simulink model "sampleModel232"  (R2021b)
settings: Solver=VariableStepAuto  StartTime=0.0  StopTime=10.0  RelTol=1e-3
undefined symbols (not defined in the file or in its folder): Newton, Raphson
libraries: simulink x12, slpidlib x3
settings Model: Creator=user  LastModifiedBy=user

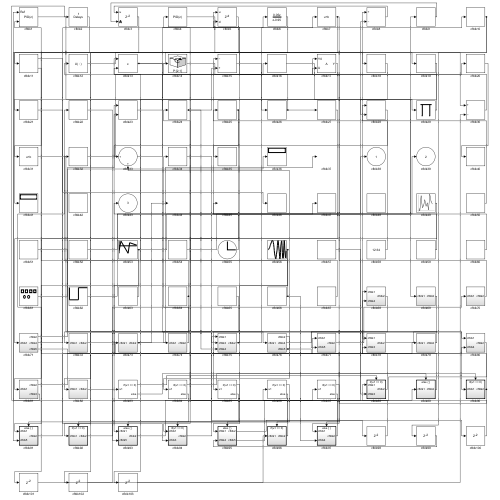
[thumbnail: Simulink's stored preview of the top-level diagram]
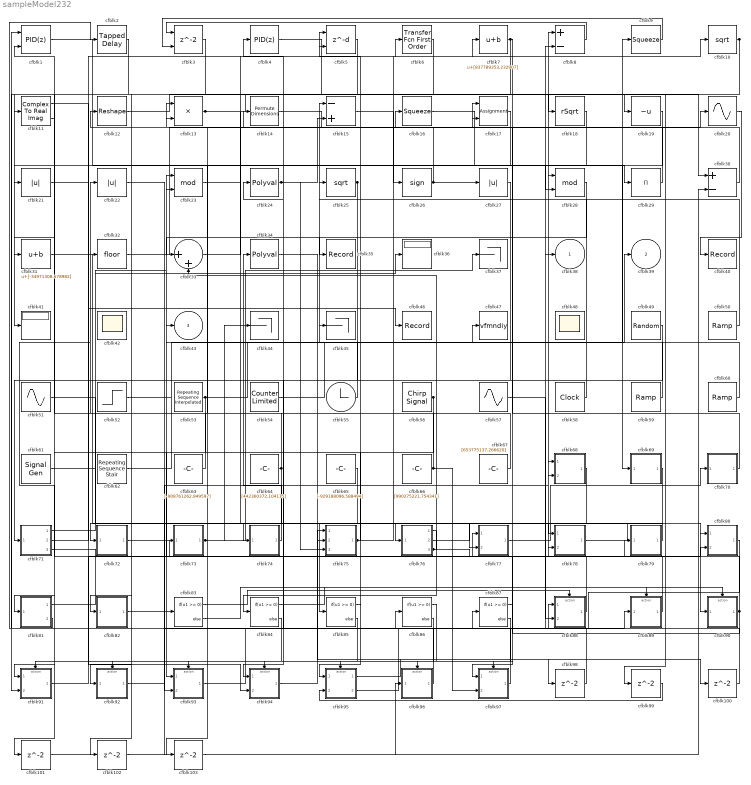
== system sampleModel232 ==
  cfblk1 : slpidlib/PID Controller (2DOF)  Controller=PID  Form=Parallel  TimeDomain=Discrete-time  UseExternalTs=off  SampleTime=1  IntegratorMethod=Forward Euler  FilterMethod=Forward Euler  ControllerParametersSource=internal  P=1  I=1  D=0  UseFilter=on  N=100  b=1  c=1  TunerSelectOption=Transfer Function Based (PID Tuner App)  InitialConditionSource=internal  InitialConditionForIntegrator=0  InitialConditionForFilter=0  DifferentiatorICPrevScaledInput=0  ExternalReset=none  TrackingMode=off  Kt=1  LimitOutput=off  SatLimitsSource=internal  UpperSaturationLimit=inf  LowerSaturationLimit=-inf  LinearizeAsGain=off  AntiWindupMode=none  Kb=1  POutMin=[]  POutMax=[]  IOutMin=[]  IOutMax=[]  DOutMin=[]  DOutMax=[]  NOutMin=[]  NOutMax=[]  bOutMin=[]  bOutMax=[]  cOutMin=[]  cOutMax=[]  SumOutMin=[]  SumOutMax=[]  SaturationOutMin=[]  SaturationOutMax=[]  PParamMin=[]  PParamMax=[]  IParamMin=[]  IParamMax=[]  DParamMin=[]  DParamMax=[]  NParamMin=[]  NParamMax=[]  bParamMin=[]  bParamMax=[]  cParamMin=[]  cParamMax=[]  KbParamMin=[]  KbParamMax=[]  KtParamMin=[]  KtParamMax=[]  KbOutMin=[]  KbOutMax=[]  KtOutMin=[]  KtOutMax=[]  IntegratorOutMin=[]  IntegratorOutMax=[]  FilterOutMin=[]  FilterOutMax=[]  SumI1OutMin=[]  SumI1OutMax=[]  SumI2OutMin=[]  SumI2OutMax=[]  SumI3OutMin=[]  SumI3OutMax=[]  SumI4OutMin=[]  SumI4OutMax=[]  SumDOutMin=[]  SumDOutMax=[]  Sum1OutMin=[]  Sum1OutMax=[]  Sum2OutMin=[]  Sum2OutMax=[]  Sum3OutMin=[]  Sum3OutMax=[]  DifferentiatorOutMin=[]  DifferentiatorOutMax=[]  FilterDiffOutCoefMin=[]  FilterDiffOutCoefMax=[]  ReciprocalOutMin=[]  ReciprocalOutMax=[]  SumDenOutMin=[]  SumDenOutMax=[]  SumNumOutMin=[]  SumNumOutMax=[]  DivideOutMin=[]  DivideOutMax=[]  UdiffTsProdOutMin=[]  UdiffTsProdOutMax=[]  NTsProdOutMin=[]  NTsProdOutMax=[]  UintegralTsProdOutMin=[]  UintegralTsProdOutMax=[]  UngainTsProdOutMin=[]  UngainTsProdOutMax=[]  IntegratorContinuousStateAttributes=''  IntegratorStateMustResolveToSignalObject=off  IntegratorRTWStateStorageClass=Auto  FilterContinuousStateAttributes=''  FilterStateMustResolveToSignalObject=off  FilterRTWStateStorageClass=Auto  ParallelPVariant=InternalParameters  IdealPVariant=Disabled  IVariant=InternalParameters  DVariant=InternalParameters  bVariant=InternalParameters  cVariant=InternalParameters  IntegratorVariant=Discrete  SatVariant=Disabled  AWVariant=Passthrough  PCopyVariant=Disabled  TRVariant=Disabled  FdbkBlocksVariant=Forward  IdealPFdbkVariant=Disabled  SatFdbkVariant=Disabled  DerivativeFilterVariant=ForwardEulerFilter  NVariant=InternalParameters  NCopyVariant=Disabled  FilterICVariant=InternalICsFilter  IntegratorICVariant=InternalICs  ExternalResetVariant=Disabled  TRSumVariant=Passthrough  SumFdbkVariant=Disabled  SumVariant=Sum_PID  TsampFilterVariant=InternalTs  TsampNgainVariant=Passthrough  TsampIntegralVariant=Passthrough  ExternalSaturationOutDataTypeStr=Inherit: Same as second input
      settings: SourceProductBaseCode=SL
  cfblk10 : Sqrt  SaturateOnIntegerOverflow=on
  cfblk{98..103} (6 alike) : Delay  SampleTime=1
  cfblk11 : ComplexToRealImag
  cfblk12 : Reshape
  cfblk13 : Product
  cfblk14 : PermuteDimensions
  cfblk15 : Sum  Inputs=-+
  cfblk16 : Squeeze
  cfblk17 : Assignment  DiagnosticForDimensions=Warning  IndexOptions=Index vector (dialog)  Indices=1  OutputSizes=1
  cfblk18 : Sqrt  Operator=rSqrt  AlgorithmType=Newton-Raphson  SaturateOnIntegerOverflow=on
  cfblk19 : UnaryMinus
  cfblk2 : simulink/Discrete/Tapped Delay  vinit=0.0  samptime=-1  NumDelays=1  DelayOrder=Oldest  includeCurrent=off
  cfblk20 : Sin  TimeSource=Use external signal  SampleTime=0
  cfblk21 : Abs
  cfblk22 : Abs
  cfblk23 : Math  Operator=mod  SaturateOnIntegerOverflow=on
  cfblk24 : Polyval  Coefs=[ +2.081618890e-019, -1.441693666e-014, +4.719686976e-010, -8.536869453e-006, +1.621573104e-001, -8.087801117e+001 ]
  cfblk25 : Sqrt  SaturateOnIntegerOverflow=on
  cfblk26 : Signum
  cfblk27 : Abs
  cfblk28 : Math  Operator=mod  SaturateOnIntegerOverflow=on
  cfblk29 : Product  Inputs=*
  cfblk3 : Delay  ShowEnablePort=on  SampleTime=1
      settings: InputPortMap=u0,e6
  cfblk30 : Sum  Inputs=+-
  cfblk31 : Bias  Bias=[-34971308.678982]
  cfblk32 : Rounding
  cfblk33 : Sum  Inputs=|++
  cfblk34 : Polyval  Coefs=[ +2.081618890e-019, -1.441693666e-014, +4.719686976e-010, -8.536869453e-006, +1.621573104e-001, -8.087801117e+001 ]
  cfblk35 : Record  FileSettingsInternal="{\"entries\":[{\"content\":{\"excelSettings\":{\"content\":{},\"type\":\"Streamout.ExcelSettings\"}},\"type\":\"Streamout.FileSettingStorage\",\"uuid\":\"16fe7588-171d-4433-9593-ebc7fb32ed17\"}],\"packageUris\":[\"http://schema.mathworks.com/mf0/streamout_blocks/R2020a\"],\"version\":\"1.0\"}"  SignalsInternal="{\"entries\":[{\"content\":{\"signals\":[{\"content\":{\"blockPath\":[\"sampleModel232/cfblk35\"],\"channel\":[],\"dimensions\":[1],\"domain\":\"sampleModel232/cfblk35\",\"lineColor\":\"#ff6929\",\"plots\":[1],\"port\":1,\"sid\":[\"\"],\"signalID\":9135,\"signalName\":\"cfblk25\"},\"type\":\"RecordBlkView.Signal\",\"uuid\":\"2eec1ae0-d335-4178-83e4-c7d2b4e411f4\"}]},\"type\":\"RecordBlkView.InputSignals\",\"uuid\":\"9f3df593-7b50-41bb-8005-8753dcf3348f\"}],\"packageUris\":[\"http://schema.mathworks.com/mf0/streamout_blocks/R2020a\"],\"version\":\"1.0\"}"  VisualizationBindings="{\"sparklinesplugin\":{\"info\":[{\"bindingParametersList\":[],\"subplotID\":1}]}}"
  cfblk36 : Display
  cfblk37 : Terminator
  cfblk4 : slpidlib/PID Controller  Controller=PID  Form=Parallel  TimeDomain=Discrete-time  UseExternalTs=off  SampleTime=1  IntegratorMethod=Forward Euler  FilterMethod=Forward Euler  ControllerParametersSource=internal  P=1  I=1  D=0  UseFilter=on  N=100  TunerSelectOption=Transfer Function Based (PID Tuner App)  InitialConditionSource=internal  InitialConditionForIntegrator=0  InitialConditionForFilter=0  DifferentiatorICPrevScaledInput=0  ExternalReset=none  TrackingMode=off  Kt=1  LimitOutput=off  SatLimitsSource=internal  UpperSaturationLimit=inf  LowerSaturationLimit=-inf  LinearizeAsGain=off  AntiWindupMode=none  Kb=1  POutMin=[]  POutMax=[]  IOutMin=[]  IOutMax=[]  DOutMin=[]  DOutMax=[]  NOutMin=[]  NOutMax=[]  SumOutMin=[]  SumOutMax=[]  SaturationOutMin=[]  SaturationOutMax=[]  PParamMin=[]  PParamMax=[]  IParamMin=[]  IParamMax=[]  DParamMin=[]  DParamMax=[]  NParamMin=[]  NParamMax=[]  KbParamMin=[]  KbParamMax=[]  KtParamMin=[]  KtParamMax=[]  KbOutMin=[]  KbOutMax=[]  KtOutMin=[]  KtOutMax=[]  IntegratorOutMin=[]  IntegratorOutMax=[]  FilterOutMin=[]  FilterOutMax=[]  SumI1OutMin=[]  SumI1OutMax=[]  SumI2OutMin=[]  SumI2OutMax=[]  SumI3OutMin=[]  SumI3OutMax=[]  SumI4OutMin=[]  SumI4OutMax=[]  SumDOutMin=[]  SumDOutMax=[]  DifferentiatorOutMin=[]  DifferentiatorOutMax=[]  FilterDiffOutCoefMin=[]  FilterDiffOutCoefMax=[]  ReciprocalOutMin=[]  ReciprocalOutMax=[]  SumDenOutMin=[]  SumDenOutMax=[]  SumNumOutMin=[]  SumNumOutMax=[]  DivideOutMin=[]  DivideOutMax=[]  UdiffTsProdOutMin=[]  UdiffTsProdOutMax=[]  NTsProdOutMin=[]  NTsProdOutMax=[]  UintegralTsProdOutMin=[]  UintegralTsProdOutMax=[]  UngainTsProdOutMin=[]  UngainTsProdOutMax=[]  IntegratorContinuousStateAttributes=''  IntegratorStateMustResolveToSignalObject=off  IntegratorRTWStateStorageClass=Auto  FilterContinuousStateAttributes=''  FilterStateMustResolveToSignalObject=off  FilterRTWStateStorageClass=Auto  ParallelPVariant=InternalParameters  IdealPVariant=Disabled  IVariant=InternalParameters  DVariant=InternalParameters  IntegratorVariant=Discrete  SatVariant=Disabled  AWVariant=Passthrough  PCopyVariant=Disabled  TRVariant=Disabled  FdbkBlocksVariant=Forward  IdealPFdbkVariant=Disabled  SatFdbkVariant=Disabled  DerivativeFilterVariant=ForwardEulerFilter  NVariant=InternalParameters  NCopyVariant=Disabled  FilterICVariant=InternalICsFilter  IntegratorICVariant=InternalICs  ExternalResetVariant=Disabled  TRSumVariant=Passthrough  SumFdbkVariant=Disabled  SumVariant=Sum_PID  TsampFilterVariant=InternalTs  TsampNgainVariant=Passthrough  TsampIntegralVariant=Passthrough  ExternalSaturationOutDataTypeStr=Inherit: Same as second input
  cfblk40 : Record  FileSettingsInternal="{\"entries\":[{\"content\":{\"excelSettings\":{\"content\":{},\"type\":\"Streamout.ExcelSettings\"}},\"type\":\"Streamout.FileSettingStorage\",\"uuid\":\"38fde572-acd1-41f4-bd4f-f8c5a046ea04\"}],\"packageUris\":[\"http://schema.mathworks.com/mf0/streamout_blocks/R2020a\"],\"version\":\"1.0\"}"  SignalsInternal="{\"entries\":[{\"content\":{\"signals\":[{\"content\":{\"blockPath\":[\"sampleModel232/cfblk40\"],\"channel\":[],\"dimensions\":[1,1],\"domain\":\"sampleModel232/cfblk40\",\"lineColor\":\"#b746ff\",\"plots\":[1],\"port\":1,\"sid\":[\"\"],\"signalID\":9139,\"signalName\":\"cfblk20\"},\"type\":\"RecordBlkView.Signal\",\"uuid\":\"00039949-2aab-479e-a4e6-845a35bec5f1\"}]},\"type\":\"RecordBlkView.InputSignals\",\"uuid\":\"6f56bbc5-1270-4389-943e-16f85e3705aa\"}],\"packageUris\":[\"http://schema.mathworks.com/mf0/streamout_blocks/R2020a\"],\"version\":\"1.0\"}"  VisualizationBindings="{\"sparklinesplugin\":{\"info\":[{\"bindingParametersList\":[],\"subplotID\":1}]}}"
  cfblk41 : Display
  cfblk42 : Scope
      settings: Floating=on
  cfblk44 : Terminator
  cfblk45 : Terminator
  cfblk46 : Record  FileSettingsInternal="{\"entries\":[{\"content\":{\"excelSettings\":{\"content\":{},\"type\":\"Streamout.ExcelSettings\"}},\"type\":\"Streamout.FileSettingStorage\",\"uuid\":\"14fcbd9d-bac8-4dc1-8b82-4cc51f23d5c0\"}],\"packageUris\":[\"http://schema.mathworks.com/mf0/streamout_blocks/R2020a\"],\"version\":\"1.0\"}"  SignalsInternal="{\"entries\":[{\"content\":{\"signals\":[{\"content\":{\"blockPath\":[\"sampleModel232/cfblk46\"],\"channel\":[],\"dimensions\":[1],\"domain\":\"sampleModel232/cfblk46\",\"lineColor\":\"#64d413\",\"plots\":[1],\"port\":1,\"sid\":[\"\"],\"signalID\":9143,\"signalName\":\"cfblk21\"},\"type\":\"RecordBlkView.Signal\",\"uuid\":\"5c7e960c-d979-495a-80ca-2dc05e47916f\"}]},\"type\":\"RecordBlkView.InputSignals\",\"uuid\":\"40783f06-613e-4da5-a4b1-e85038e253b6\"}],\"packageUris\":[\"http://schema.mathworks.com/mf0/streamout_blocks/R2020a\"],\"version\":\"1.0\"}"  VisualizationBindings="{\"sparklinesplugin\":{\"info\":[{\"bindingParametersList\":[],\"subplotID\":1}]}}"
  cfblk47 : ToWorkspace  VariableName=vfmndiy  SaveFormat=Timeseries  SampleTime=-1
  cfblk48 : Scope
      settings: Floating=on
  cfblk49 : UniformRandomNumber  Minimum=[-6531070159.920979]  Maximum=[9416126796.491138]  Seed=[69575523.000000]  SampleTime=0.1
  cfblk5 : Delay  DelayLengthSource=Input port  SampleTime=1
      settings: InputPortMap=u0,p1
  cfblk50 : simulink/Sources/Ramp  slope=[4184.454885]  start=[6.485913]  InitialOutput=[-74727.507145]
  cfblk51 : Sin  Amplitude=[660836830.199607]  Bias=[-337757806.375018]  SampleTime=0
  cfblk52 : Step  Time=[5.000000]  Before=[-35343837.291775]  After=[252133215.622026]  SampleTime=0
  cfblk53 : simulink/Sources/Repeating Sequence Interpolated  OutValues=[-608474345.099651, 600750965.712178, -937019260.295574, 395421429.511669, 62724602.129927]  TimeValues=[0 0.1 0.5 0.6 1].'  LookUpMeth=Use Input Nearest  tsamp=0.01  OutMin=[]  OutMax=[]  OutDataTypeStr=double  OutputDataTypeScalingMode=double  OutDataType=fixdt(0,8)  OutScaling=2^-10
  cfblk54 : simulink/Sources/Counter Limited  uplimit=[972.000000]  tsamp=-1
  cfblk55 : Clock
  cfblk56 : simulink/Sources/Chirp Signal  f1=[693040230.893386]  T=[-954068434.723357]  f2=[440264525.580880]
  cfblk57 : Sin  Amplitude=[242398372.769042]  Bias=[-91557625.579191]  SampleTime=0
  cfblk58 : DigitalClock
  cfblk59 : simulink/Sources/Ramp  slope=[-2546.341926]  start=[42.940837]  InitialOutput=[85456.918495]
  cfblk6 : simulink/Discrete/Transfer Fcn First Order  PoleZ=0.95  ICPrevOutput=0.0  DoSatur=off
  cfblk60 : simulink/Sources/Ramp  slope=[-9968.943757]  start=[29.827868]  InitialOutput=[-927129.818400]
  cfblk61 : SignalGenerator  WaveForm=square  Amplitude=[-206501216.018369]
  cfblk62 : simulink/Sources/Repeating Sequence Stair  OutValues=[-478930033.945131, -287515944.626940]  tsamp=-1  OutMin=[]  OutMax=[]  OutDataTypeStr=double  OutputDataTypeScalingMode=double  OutDataType=fixdt(0,8)  ConRadixGroup=Best Precision: Vector-wise  OutScaling=2^-12
  cfblk63 : Constant  Value=[-908761262.849597]  SampleTime=1
  cfblk64 : Constant  Value=[442360372.104115]  SampleTime=1
  cfblk65 : Constant  Value=[-929188096.588494]  SampleTime=1
  cfblk66 : Constant  Value=[990275221.754341]  SampleTime=1
  cfblk67 : Constant  Value=[653775137.266620]  SampleTime=1
  cfblk68 : Subsystem
  cfblk69 : Subsystem
  cfblk7 : Bias  Bias=[837789353.232907]
  cfblk70 : Subsystem
  cfblk71 : Subsystem
  cfblk72 : Subsystem
  cfblk73 : Subsystem
  cfblk74 : Subsystem
  cfblk75 : Subsystem
  cfblk76 : Subsystem
  cfblk77 : Subsystem
  cfblk78 : Subsystem
  cfblk79 : Subsystem
  cfblk8 : Sum  Inputs=+-
  cfblk80 : Subsystem
  cfblk81 : Subsystem
  cfblk82 : Subsystem
  cfblk{83..87} (5 alike) : If  IfExpression=u1 >= 0  SampleTime=1
  cfblk88 : Subsystem  TreatAsAtomicUnit=on
  cfblk89 : Subsystem  TreatAsAtomicUnit=on
  cfblk9 : Squeeze
  cfblk90 : Subsystem  TreatAsAtomicUnit=on
  cfblk91 : Subsystem  TreatAsAtomicUnit=on
  cfblk92 : Subsystem  TreatAsAtomicUnit=on
  cfblk93 : Subsystem  TreatAsAtomicUnit=on
  cfblk94 : Subsystem  TreatAsAtomicUnit=on
  cfblk95 : Subsystem  TreatAsAtomicUnit=on
  cfblk96 : Subsystem  TreatAsAtomicUnit=on
  cfblk97 : Subsystem  TreatAsAtomicUnit=on
  cfblk38 : Outport
  cfblk39 : Outport  Port=2
  cfblk43 : Outport  Port=3
  wires:
  cfblk32/1 -> cfblk16/1
  cfblk61/1 -> cfblk36/1
  cfblk93/1(cfblk2) -> cfblk87/1
  cfblk88/1(cfblk2) -> cfblk8/1
  cfblk80/1(cfblk2) -> cfblk88/1(cfblk1)
  cfblk79/1(cfblk2) -> cfblk72/1(cfblk1)
  cfblk12/1 -> cfblk18/1
  cfblk50/1 -> cfblk15/1
  cfblk90/1(cfblk2) -> cfblk22/1, cfblk78/2(cfblk3)
  cfblk51/1 -> cfblk90/1(cfblk1)
  cfblk89/1(cfblk2) -> cfblk23/1
  cfblk14/1 -> cfblk20/1
  cfblk17/1 -> cfblk41/1
  cfblk27/1 -> cfblk71/1(cfblk1)
  cfblk54/1 -> cfblk8/2
  cfblk52/1 -> cfblk47/1
  cfblk8/1 -> cfblk3/1
  cfblk64/1 -> cfblk92/1(cfblk1), cfblk1/2
  cfblk53/1 -> cfblk93/1(cfblk1), cfblk39/1
  cfblk74/1(cfblk2) -> cfblk34/1
  cfblk97/1(cfblk2) -> cfblk24/1
  cfblk26/1 -> cfblk27/1, cfblk5/1
  cfblk65/1 -> cfblk85/1
  cfblk60/1 -> cfblk25/1
  cfblk92/1(cfblk2) -> cfblk89/1(cfblk1)
  cfblk15/1 -> cfblk26/1
  cfblk24/1 -> cfblk15/2, cfblk75/3(cfblk4)
  cfblk31/1 -> cfblk76/1(cfblk1)
  cfblk7/1 -> cfblk21/1, cfblk97/1(cfblk1)
  cfblk4/1 -> cfblk30/1
  cfblk55/1 -> cfblk45/1
  cfblk66/1 -> cfblk4/1, cfblk97/2(cfblk4)
  cfblk56/1 -> cfblk91/1(cfblk1), cfblk95/1(cfblk1)
  cfblk78/1(cfblk2) -> cfblk80/1(cfblk1)
  cfblk21/1 -> cfblk46/1
  cfblk20/1 -> cfblk40/1
  cfblk33/1 -> cfblk7/1
  cfblk13/1 -> cfblk19/1, cfblk75/2(cfblk3)
  cfblk1/1 -> cfblk29/1
  cfblk30/1 -> cfblk12/1
  cfblk57/1 -> cfblk88/2(cfblk3)
  cfblk81/1(cfblk2) -> cfblk68/1(cfblk1)
  cfblk96/1(cfblk2) -> cfblk14/1
  cfblk91/1(cfblk2) -> cfblk77/1(cfblk1)
  cfblk75/1(cfblk2) -> cfblk10/1, cfblk5/2
  cfblk73/1(cfblk2) -> cfblk37/1, cfblk44/1
  cfblk94/1(cfblk2) -> cfblk75/1(cfblk1)
  cfblk58/1 -> cfblk28/1
  cfblk81/2(cfblk3) -> cfblk2/1
  cfblk71/1(cfblk2) -> cfblk23/2
  cfblk9/1 -> cfblk3/2
  cfblk76/1(cfblk2) -> cfblk84/1
  cfblk5/1 -> cfblk91/2(cfblk5)
  cfblk6/1 -> cfblk11/1
  cfblk77/1(cfblk2) -> cfblk70/1(cfblk1)
  cfblk68/1(cfblk2) -> cfblk74/1(cfblk1)
  cfblk63/1 -> cfblk32/1
  cfblk82/1(cfblk2) -> cfblk68/2(cfblk4)
  cfblk25/1 -> cfblk81/1(cfblk1), cfblk35/1
  cfblk16/1 -> cfblk69/1(cfblk1)
  cfblk62/1 -> cfblk9/1
  cfblk49/1 -> cfblk94/1(cfblk1)
  cfblk67/1 -> cfblk13/1
  cfblk59/1 -> cfblk43/1
  cfblk22/1 -> cfblk93/2(cfblk5)
  cfblk10/1 -> cfblk82/1(cfblk1), cfblk99/1
  cfblk2/1 -> cfblk31/1
  cfblk69/1(cfblk2) -> cfblk77/2(cfblk5)
  cfblk11/1 -> cfblk94/2(cfblk3)
  cfblk19/1 -> cfblk28/2
  cfblk95/2(cfblk5) -> cfblk38/1
  cfblk76/2(cfblk4) -> cfblk78/1(cfblk1)
  cfblk29/1 -> cfblk13/2
  cfblk70/1(cfblk2) -> cfblk17/1
  cfblk76/3(cfblk5) -> cfblk79/1(cfblk1), cfblk33/2
  cfblk72/1(cfblk2) -> cfblk80/2(cfblk4)
  cfblk23/1 -> cfblk17/2
  cfblk71/2(cfblk4) -> cfblk6/1
  cfblk28/1 -> cfblk33/1
  cfblk71/3(cfblk5) -> cfblk73/1(cfblk1)
  cfblk83/1 -> cfblk88/Action
  cfblk83/2 -> cfblk89/Action
  cfblk84/1 -> cfblk90/Action
  cfblk84/2 -> cfblk91/Action
  cfblk85/1 -> cfblk92/Action
  cfblk85/2 -> cfblk93/Action
  cfblk86/1 -> cfblk94/Action
  cfblk86/2 -> cfblk95/Action
  cfblk87/1 -> cfblk96/Action
  cfblk87/2 -> cfblk97/Action
  cfblk34/1 -> cfblk98/1
  cfblk98/1 -> cfblk1/1
  cfblk99/1 -> cfblk95/2(cfblk4)
  cfblk95/1(cfblk2) -> cfblk100/1
  cfblk100/1 -> cfblk86/1
  cfblk11/2 -> cfblk101/1
  cfblk101/1 -> cfblk96/1(cfblk1)
  cfblk3/1 -> cfblk102/1
  cfblk102/1 -> cfblk83/1
  cfblk18/1 -> cfblk103/1
  cfblk103/1 -> cfblk30/2

== system sampleModel232/cfblk68 ==
  cfblk1 : Inport
  cfblk4 : Inport  Port=2
  cfblk3 : simulink/Discrete/Tapped Delay  vinit=0.0  samptime=-1  NumDelays=1  DelayOrder=Oldest  includeCurrent=off
  cfblk2 : Outport
  wires:
  cfblk1/1 -> cfblk3/1
  cfblk3/1 -> cfblk2/1

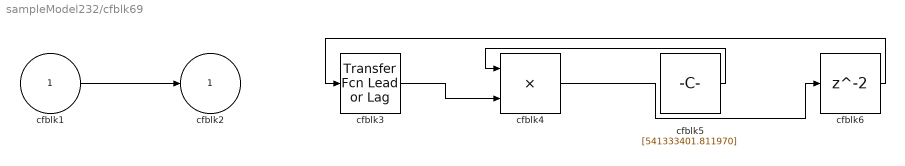
== system sampleModel232/cfblk69 ==
  cfblk1 : Inport
  cfblk3 : simulink/Discrete/Transfer Fcn Lead or Lag  PoleZ=0.95  ZeroZ=0.75  ICPrevOutput=0.0  ICPrevInput=0.0  DoSatur=off
      settings: SourceProductBaseCode=SL
  cfblk4 : Product
  cfblk5 : Constant  Value=[541333401.811970]  SampleTime=1
  cfblk6 : Delay  SampleTime=1
  cfblk2 : Outport
  wires:
  cfblk5/1 -> cfblk4/1
  cfblk1/1 -> cfblk2/1
  cfblk3/1 -> cfblk4/2
  cfblk4/1 -> cfblk6/1
  cfblk6/1 -> cfblk3/1

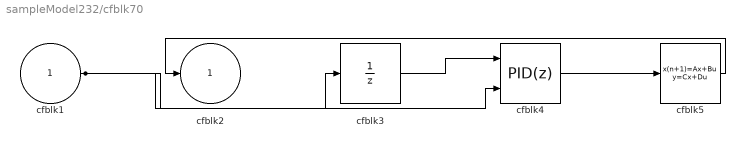
== system sampleModel232/cfblk70 ==
  cfblk1 : Inport
  cfblk3 : UnitDelay  HasFrameUpgradeWarning=on
  cfblk4 : slpidlib/PID Controller (2DOF)  Controller=PID  Form=Parallel  TimeDomain=Discrete-time  UseExternalTs=off  SampleTime=1  IntegratorMethod=Forward Euler  FilterMethod=Forward Euler  ControllerParametersSource=internal  P=1  I=1  D=0  UseFilter=on  N=100  b=1  c=1  TunerSelectOption=Transfer Function Based (PID Tuner App)  InitialConditionSource=internal  InitialConditionForIntegrator=0  InitialConditionForFilter=0  DifferentiatorICPrevScaledInput=0  ExternalReset=none  TrackingMode=off  Kt=1  LimitOutput=off  SatLimitsSource=internal  UpperSaturationLimit=inf  LowerSaturationLimit=-inf  LinearizeAsGain=off  AntiWindupMode=none  Kb=1  POutMin=[]  POutMax=[]  IOutMin=[]  IOutMax=[]  DOutMin=[]  DOutMax=[]  NOutMin=[]  NOutMax=[]  bOutMin=[]  bOutMax=[]  cOutMin=[]  cOutMax=[]  SumOutMin=[]  SumOutMax=[]  SaturationOutMin=[]  SaturationOutMax=[]  PParamMin=[]  PParamMax=[]  IParamMin=[]  IParamMax=[]  DParamMin=[]  DParamMax=[]  NParamMin=[]  NParamMax=[]  bParamMin=[]  bParamMax=[]  cParamMin=[]  cParamMax=[]  KbParamMin=[]  KbParamMax=[]  KtParamMin=[]  KtParamMax=[]  KbOutMin=[]  KbOutMax=[]  KtOutMin=[]  KtOutMax=[]  IntegratorOutMin=[]  IntegratorOutMax=[]  FilterOutMin=[]  FilterOutMax=[]  SumI1OutMin=[]  SumI1OutMax=[]  SumI2OutMin=[]  SumI2OutMax=[]  SumI3OutMin=[]  SumI3OutMax=[]  SumI4OutMin=[]  SumI4OutMax=[]  SumDOutMin=[]  SumDOutMax=[]  Sum1OutMin=[]  Sum1OutMax=[]  Sum2OutMin=[]  Sum2OutMax=[]  Sum3OutMin=[]  Sum3OutMax=[]  DifferentiatorOutMin=[]  DifferentiatorOutMax=[]  FilterDiffOutCoefMin=[]  FilterDiffOutCoefMax=[]  ReciprocalOutMin=[]  ReciprocalOutMax=[]  SumDenOutMin=[]  SumDenOutMax=[]  SumNumOutMin=[]  SumNumOutMax=[]  DivideOutMin=[]  DivideOutMax=[]  UdiffTsProdOutMin=[]  UdiffTsProdOutMax=[]  NTsProdOutMin=[]  NTsProdOutMax=[]  UintegralTsProdOutMin=[]  UintegralTsProdOutMax=[]  UngainTsProdOutMin=[]  UngainTsProdOutMax=[]  IntegratorContinuousStateAttributes=''  IntegratorStateMustResolveToSignalObject=off  IntegratorRTWStateStorageClass=Auto  FilterContinuousStateAttributes=''  FilterStateMustResolveToSignalObject=off  FilterRTWStateStorageClass=Auto  ParallelPVariant=InternalParameters  IdealPVariant=Disabled  IVariant=InternalParameters  DVariant=InternalParameters  bVariant=InternalParameters  cVariant=InternalParameters  IntegratorVariant=Discrete  SatVariant=Disabled  AWVariant=Passthrough  PCopyVariant=Disabled  TRVariant=Disabled  FdbkBlocksVariant=Forward  IdealPFdbkVariant=Disabled  SatFdbkVariant=Disabled  DerivativeFilterVariant=ForwardEulerFilter  NVariant=InternalParameters  NCopyVariant=Disabled  FilterICVariant=InternalICsFilter  IntegratorICVariant=InternalICs  ExternalResetVariant=Disabled  TRSumVariant=Passthrough  SumFdbkVariant=Disabled  SumVariant=Sum_PID  TsampFilterVariant=InternalTs  TsampNgainVariant=Passthrough  TsampIntegralVariant=Passthrough  ExternalSaturationOutDataTypeStr=Inherit: Same as second input
      settings: SourceProductBaseCode=SL
  cfblk5 : DiscreteStateSpace
  cfblk2 : Outport
  wires:
  cfblk5/1 -> cfblk2/1
  cfblk1/1 -> cfblk3/1, cfblk4/2
  cfblk3/1 -> cfblk4/1
  cfblk4/1 -> cfblk5/1

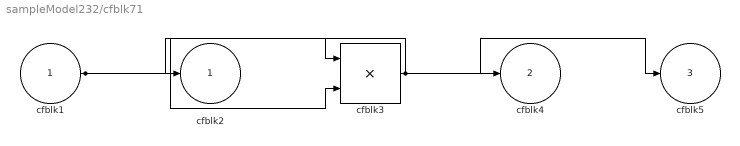
== system sampleModel232/cfblk71 ==
  cfblk1 : Inport
  cfblk3 : Product
  cfblk2 : Outport
  cfblk4 : Outport  Port=2
  cfblk5 : Outport  Port=3
  wires:
  cfblk3/1 -> cfblk4/1, cfblk2/1, cfblk5/1
  cfblk1/1 -> cfblk3/1, cfblk3/2

== system sampleModel232/cfblk72 ==
  cfblk1 : Inport
  cfblk3 : Delay  SampleTime=1
  cfblk2 : Outport
  wires:
  cfblk1/1 -> cfblk3/1
  cfblk3/1 -> cfblk2/1

== system sampleModel232/cfblk73 ==
  cfblk1 : Inport
  cfblk3 : Delay  ShowEnablePort=on  SampleTime=1
      settings: InputPortMap=u0,e6
  cfblk4 : Sqrt  SaturateOnIntegerOverflow=on
  cfblk2 : Outport
  wires:
  cfblk1/1 -> cfblk4/1, cfblk3/2
  cfblk4/1 -> cfblk3/1
  cfblk3/1 -> cfblk2/1

== system sampleModel232/cfblk74 ==
  cfblk1 : Inport
  cfblk3 : Constant  Value=[667065563.085386]  SampleTime=1
  cfblk2 : Outport
  wires:
  cfblk1/1 -> cfblk2/1

== system sampleModel232/cfblk75 ==
  cfblk1 : Inport
  cfblk3 : Inport  Port=2
  cfblk4 : Inport  Port=3
  cfblk2 : Outport
  wires:
  cfblk1/1 -> cfblk2/1

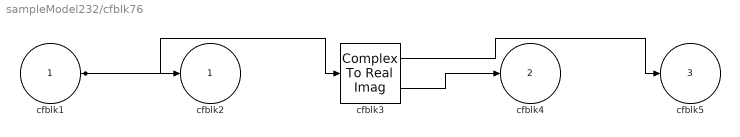
== system sampleModel232/cfblk76 ==
  cfblk1 : Inport
  cfblk3 : ComplexToRealImag
  cfblk2 : Outport
  cfblk4 : Outport  Port=2
  cfblk5 : Outport  Port=3
  wires:
  cfblk3/1 -> cfblk5/1
  cfblk1/1 -> cfblk2/1, cfblk3/1
  cfblk3/2 -> cfblk4/1

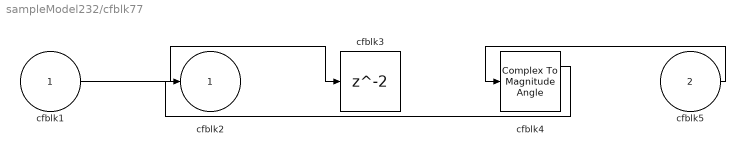
== system sampleModel232/cfblk77 ==
  cfblk1 : Inport
  cfblk5 : Inport  Port=2
  cfblk3 : Delay  SampleTime=1
  cfblk4 : ComplexToMagnitudeAngle
  cfblk2 : Outport
  wires:
  cfblk5/1 -> cfblk4/1
  cfblk1/1 -> cfblk3/1
  cfblk4/1 -> cfblk2/1

== system sampleModel232/cfblk78 ==
  cfblk1 : Inport
  cfblk3 : Inport  Port=2
  cfblk2 : Outport
  wires:
  cfblk3/1 -> cfblk2/1

== system sampleModel232/cfblk79 ==
  cfblk1 : Inport
  cfblk3 : Rounding
  cfblk2 : Outport
  wires:
  cfblk3/1 -> cfblk2/1
  cfblk1/1 -> cfblk3/1

== system sampleModel232/cfblk80 ==
  cfblk1 : Inport
  cfblk4 : Inport  Port=2
  cfblk3 : Delay  SampleTime=1
  cfblk2 : Outport
  wires:
  cfblk4/1 -> cfblk3/1
  cfblk1/1 -> cfblk2/1

== system sampleModel232/cfblk81 ==
  cfblk1 : Inport
  cfblk2 : Outport
  cfblk3 : Outport  Port=2
  wires:
  cfblk1/1 -> cfblk3/1, cfblk2/1

== system sampleModel232/cfblk82 ==
  cfblk1 : Inport
  cfblk3 : Sum  Inputs=+
  cfblk4 : Sum  Inputs=+
  cfblk2 : Outport
  wires:
  cfblk1/1 -> cfblk4/1
  cfblk3/1 -> cfblk2/1
  cfblk4/1 -> cfblk3/1

== system sampleModel232/cfblk88 ==
  cfblk1 : Inport
  cfblk3 : Inport  Port=2
  Action Port : ActionPort  ActionPortLabel=if(u1 >= 0)
  cfblk2 : Outport
  wires:
  cfblk1/1 -> cfblk2/1

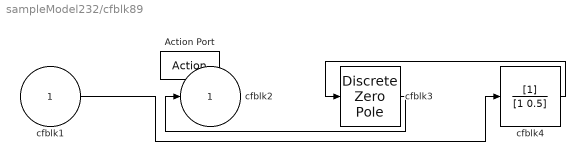
== system sampleModel232/cfblk89 ==
  cfblk1 : Inport
  Action Port : ActionPort  ActionPortLabel=else
  cfblk3 : DiscreteZeroPole  Poles=[0 0.5]  Gain=1  SampleTime=-1
  cfblk4 : DiscreteFilter
  cfblk2 : Outport
  wires:
  cfblk3/1 -> cfblk2/1
  cfblk1/1 -> cfblk4/1
  cfblk4/1 -> cfblk3/1

== system sampleModel232/cfblk90 ==
  cfblk1 : Inport
  Action Port : ActionPort  ActionPortLabel=if(u1 >= 0)
  cfblk3 : simulink/Discrete/Transfer Fcn Lead or Lag  PoleZ=0.95  ZeroZ=0.75  ICPrevOutput=0.0  ICPrevInput=0.0  DoSatur=off
      settings: SourceProductBaseCode=SL
  cfblk2 : Outport
  wires:
  cfblk1/1 -> cfblk2/1, cfblk3/1

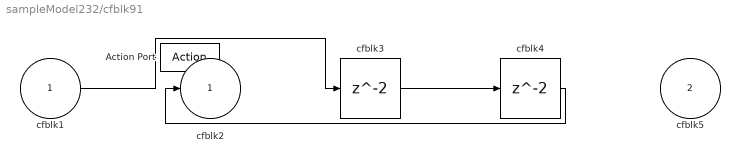
== system sampleModel232/cfblk91 ==
  cfblk1 : Inport
  cfblk5 : Inport  Port=2
  Action Port : ActionPort  ActionPortLabel=else
  cfblk3 : Delay
  cfblk4 : Delay
  cfblk2 : Outport
  wires:
  cfblk3/1 -> cfblk4/1
  cfblk4/1 -> cfblk2/1
  cfblk1/1 -> cfblk3/1

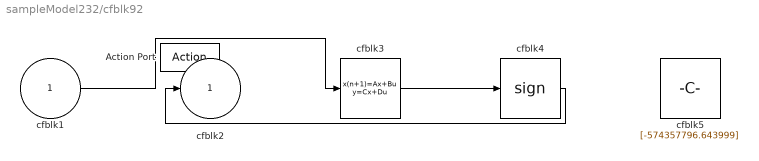
== system sampleModel232/cfblk92 ==
  cfblk1 : Inport
  Action Port : ActionPort  ActionPortLabel=if(u1 >= 0)
  cfblk3 : DiscreteStateSpace  SampleTime=-1
  cfblk4 : Signum
  cfblk5 : Constant  Value=[-574357796.643999]  SampleTime=1
  cfblk2 : Outport
  wires:
  cfblk4/1 -> cfblk2/1
  cfblk1/1 -> cfblk3/1
  cfblk3/1 -> cfblk4/1

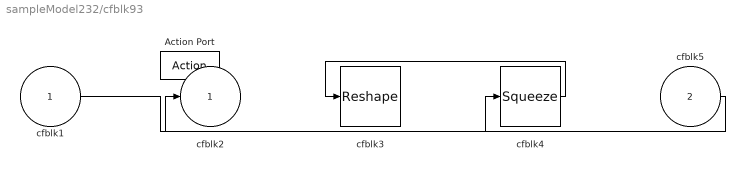
== system sampleModel232/cfblk93 ==
  cfblk1 : Inport
  cfblk5 : Inport  Port=2
  Action Port : ActionPort  ActionPortLabel=else
  cfblk3 : Reshape
  cfblk4 : Squeeze
  cfblk2 : Outport
  wires:
  cfblk5/1 -> cfblk2/1
  cfblk4/1 -> cfblk3/1
  cfblk1/1 -> cfblk4/1

== system sampleModel232/cfblk94 ==
  cfblk1 : Inport
  cfblk3 : Inport  Port=2
  Action Port : ActionPort  ActionPortLabel=if(u1 >= 0)
  cfblk2 : Outport
  wires:
  cfblk1/1 -> cfblk2/1

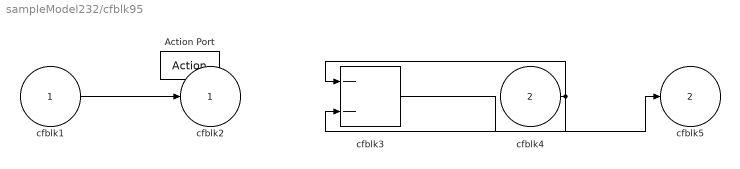
== system sampleModel232/cfblk95 ==
  cfblk1 : Inport
  cfblk4 : Inport  Port=2
  Action Port : ActionPort  ActionPortLabel=else
  cfblk3 : Sum  Inputs=--
  cfblk2 : Outport
  cfblk5 : Outport  Port=2
  wires:
  cfblk4/1 -> cfblk3/1, cfblk3/2
  cfblk3/1 -> cfblk5/1
  cfblk1/1 -> cfblk2/1

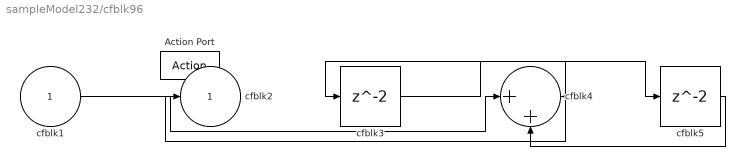
== system sampleModel232/cfblk96 ==
  cfblk1 : Inport
  Action Port : ActionPort  ActionPortLabel=if(u1 >= 0)
  cfblk3 : Delay
  cfblk4 : Sum  Inputs=|++
  cfblk5 : Delay
  cfblk2 : Outport
  wires:
  cfblk1/1 -> cfblk4/1
  cfblk4/1 -> cfblk2/1, cfblk3/1
  cfblk3/1 -> cfblk5/1
  cfblk5/1 -> cfblk4/2

== system sampleModel232/cfblk97 ==
  cfblk1 : Inport
  cfblk4 : Inport  Port=2
  Action Port : ActionPort  ActionPortLabel=else
  cfblk3 : Constant  Value=[-863625591.593459]  SampleTime=1
  cfblk2 : Outport
  wires:
  cfblk1/1 -> cfblk2/1
